simulink model "rohr_2"  (Simulink 4.00)
settings: Solver=ode23s  StartTime=0.0  StopTime=200  MaxStep=0.1  RelTol=10e-3
values from neighbouring files (symbols this model uses):
  A = zeros(10,10);			A(1:5,6:10) = eye(5,5)    [mehrw_1.m]    (also in mehrw_2.m; mehrw_3.m; mehrw_4.m; mehrw_5.m)
  b = 1    [anw_pid_1.m]    (also in mehrw_4.m = my_system1.b; mehrw_5.m = my_system1.b)
  g = 9.81    [behaelter_1.m]    (also in behaelter_2.m; kette_1.m = 9.8; pendel_1.m = 9.8; pendel_2.m = 9.8)
  h0 = m0/(ro*AB)    (= 0.707355302631)    [behaelter_1.m]    (also in behaelter_2.m)
  l = 1    [pendel_1.m]
  r = 2    [behaelter_1.m]    (also in behaelter_2.m; mehrw_1.m = [0.05, 0.05, 0.05, 0.05, 0.05]; mehrw_2.m = [0.05, 0.05, 0.05, 0.05, 0.05]; mehrw_3.m = [0.05, 0.05, 0.05, 0.05, 0.05])
undefined symbols (not defined in the file or in its folder): freq, omega_final, step_v
settings Model: LastModifiedBy=Administrator  Refine=5  BlockReductionOpt=off

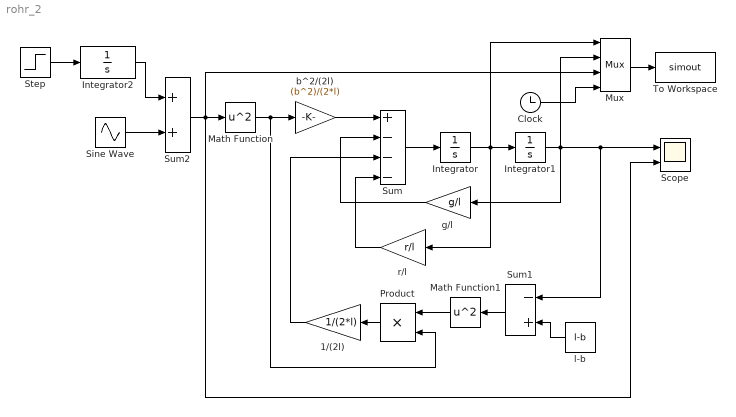
== system rohr_2 ==
  1/(2l) : Gain  Orientation=left  Gain=1/(2*l)  Multiplication=Element-wise(K.*u)  SaturateOnIntegerOverflow=on
  Clock : Clock
      settings: DisplayTime=off  Decimation=10
  Integrator : Integrator  ExternalReset=none  InitialConditionSource=internal  InitialCondition=0  LimitOutput=off  UpperSaturationLimit=inf  LowerSaturationLimit=-inf  ShowSaturationPort=off  ShowStatePort=off  AbsoluteTolerance=auto
  Integrator1 : Integrator  ExternalReset=none  InitialConditionSource=internal  InitialCondition=h0  LimitOutput=off  UpperSaturationLimit=inf  LowerSaturationLimit=-inf  ShowSaturationPort=off  ShowStatePort=off  AbsoluteTolerance=auto
  Integrator2 : Integrator  ExternalReset=none  InitialConditionSource=internal  InitialCondition=0  LimitOutput=on  UpperSaturationLimit=omega_final  LowerSaturationLimit=0  ShowSaturationPort=off  ShowStatePort=off  AbsoluteTolerance=auto
  Math Function : Math  Operator=square  OutputSignalType=auto
  Math Function1 : Math  Orientation=left  Operator=square  OutputSignalType=auto
  Mux : Mux  Inputs=4
      settings: DisplayOption=none
  Product : Product  Orientation=left  Inputs=2  Multiplication=Element-wise(.*)  SaturateOnIntegerOverflow=on
  Scope : Scope  NumInputPorts=2
      settings: TimeRange=auto  YMin=0~-3  YMax=10~5  SaveToWorkspace=off  SaveName=ScopeData  MaxDataPoints=5000
  Sine Wave : Sin  Amplitude=A  Frequency=2*pi*freq  Phase=0  SampleTime=0
  Step : Step  Time=0  Before=0  After=step_v  SampleTime=0
  Sum : Sum  Inputs=+---  SaturateOnIntegerOverflow=on
  Sum1 : Sum  Orientation=left  Inputs=-+  SaturateOnIntegerOverflow=on
  Sum2 : Sum  Inputs=++  SaturateOnIntegerOverflow=on
  To Workspace : ToWorkspace  VariableName=simout  SampleTime=-1  SaveFormat=Array
  b^2/(2l) : Gain  Gain=(b^2)/(2*l)  Multiplication=Element-wise(K.*u)  SaturateOnIntegerOverflow=on
  g/l : Gain  Orientation=left  Gain=g/l  Multiplication=Element-wise(K.*u)  SaturateOnIntegerOverflow=on
  l-b : Constant  Orientation=left  Value=l-b
  r/l : Gain  Orientation=left  Gain=r/l  Multiplication=Element-wise(K.*u)  SaturateOnIntegerOverflow=on
  wires:
  Math Function/1 -> b^2/(2l)/1, Product/2
  b^2/(2l)/1 -> Sum/1
  Sum/1 -> Integrator/1
  Integrator/1 -> Integrator1/1, r/l/1, Mux/1
  Integrator1/1 -> Sum1/1, Scope/1, g/l/1, Mux/2
  l-b/1 -> Sum1/2
  Sum1/1 -> Math Function1/1
  Math Function1/1 -> Product/1
  Product/1 -> 1/(2l)/1
  1/(2l)/1 -> Sum/3
  g/l/1 -> Sum/2
  r/l/1 -> Sum/4
  Mux/1 -> To Workspace/1
  Clock/1 -> Mux/4
  Step/1 -> Integrator2/1
  Sum2/1 -> Math Function/1, Scope/2, Mux/3
  Sine Wave/1 -> Sum2/2
  Integrator2/1 -> Sum2/1
